simulink model "Demo_veDYNA_cs"  (Simulink 7.6)
settings: Solver=ode1  StartTime=0  StopTime=15  FixedStep=1/500  RelTol=1e-3
PreLoadFcn:
  | PreScanveDYNAPreLoadFcn(bdroot);
  | check_NUTS_defined;
  | 
  | assignin('base',['model_closed_' bdroot],false);
PostLoadFcn:
  | PreScanveDYNAPostLoadFcn(bdroot);
  | 
InitFcn:
  | vdy_SetExternalInputSource('ManLongCtrl',1,'Brake','other');
  | vdy_SetExternalInputSource('ManLongCtrl',1,'EngineTorque','other');
  | vdy_SetExternalInputSource('ManLatCtrl',1,'Steering','other');
  | 
  | PreScanveDYNAInitFcn(bdroot);
  | PreScanExperimentInitFcn(bdroot)
StopFcn:
  | PreScanExperimentStopFcn(bdroot)
undefined symbols (not defined in the file): at_period, CPT, vm_at_pulsewidth, vm_driver_dflt_gain, x_ini_VRML, y_ini_VRML, z_ini_VRML
libraries: dyna_cpt_lib x93, simulink x16, simulink_extras x14, PreScanSimulinkLibrary x6, anilib x3, dyna_lib x3, dyna_manctrl_lib x2, dyna_road_lib x2, PreScanUsefulBlocks x1, dyna_io_lib x1, dyna_demo_lib x1, dyna_usr_maneuver_states_lib x1
(part 8 of 8)

== system Demo_veDYNA_cs/Vedyna_Vehicle/CPT_MDL/MDL_SW/Driver/System Instance 1/lat_for_r_sw [1,..,4] ==
  Switch : Constant  Value=CPT.MDL_SW.Driver{1}.lat_for_r_sw.Switch.v
  Terminator : Terminator
  tag scope: Driver_1_lat_for_r_sw_SW=global
  wires:
  [Driver_1_lat_for_r_sw_SW] -> Terminator/1
  Switch/1 -> [Driver_1_lat_for_r_sw_SW]

== system Demo_veDYNA_cs/Vedyna_Vehicle/CPT_MDL/MDL_SW/Driver/System Instance 1/path_v_scale [1,..,4] ==
  Switch : Constant  Value=CPT.MDL_SW.Driver{1}.path_v_scale.Switch.v
  Terminator : Terminator
  tag scope: Driver_1_path_v_scale_SW=global
  wires:
  [Driver_1_path_v_scale_SW] -> Terminator/1
  Switch/1 -> [Driver_1_path_v_scale_SW]

== system Demo_veDYNA_cs/Vedyna_Vehicle/CPT_MDL/MDL_SW/Driver/System Instance 1/path_x_offset [1,..,4] ==
  Switch : Constant  Value=CPT.MDL_SW.Driver{1}.path_x_offset.Switch.v
  Terminator : Terminator
  tag scope: Driver_1_path_x_offset_SW=global
  wires:
  [Driver_1_path_x_offset_SW] -> Terminator/1
  Switch/1 -> [Driver_1_path_x_offset_SW]

== system Demo_veDYNA_cs/Vedyna_Vehicle/CPT_MDL/MDL_SW/Driver/System Instance 1/psi_path [1,..,4] ==
  Switch : Constant  Value=CPT.MDL_SW.Driver{1}.psi_path.Switch.v
  Terminator : Terminator
  tag scope: Driver_1_psi_path_SW=global
  wires:
  [Driver_1_psi_path_SW] -> Terminator/1
  Switch/1 -> [Driver_1_psi_path_SW]

== system Demo_veDYNA_cs/Vedyna_Vehicle/CPT_MDL/MDL_SW/Driver/System Instance 1/q_path [1,..,4] ==
  Switch : Constant  Value=CPT.MDL_SW.Driver{1}.q_path.Switch.v
  Terminator : Terminator
  tag scope: Driver_1_q_path_SW=global
  wires:
  [Driver_1_q_path_SW] -> Terminator/1
  Switch/1 -> [Driver_1_q_path_SW]

== system Demo_veDYNA_cs/Vedyna_Vehicle/CPT_MDL/MDL_SW/Driver/System Instance 1/rear_stiff [1,..,4] ==
  Switch : Constant  Value=CPT.MDL_SW.Driver{1}.rear_stiff.Switch.v
  Terminator : Terminator
  tag scope: Driver_1_rear_stiff_SW=global
  wires:
  [Driver_1_rear_stiff_SW] -> Terminator/1
  Switch/1 -> [Driver_1_rear_stiff_SW]

== system Demo_veDYNA_cs/Vedyna_Vehicle/CPT_MDL/MDL_SW/Driver/System Instance 1/rear_stiff_sw [1,..,4] ==
  Switch : Constant  Value=CPT.MDL_SW.Driver{1}.rear_stiff_sw.Switch.v
  Terminator : Terminator
  tag scope: Driver_1_rear_stiff_sw_SW=global
  wires:
  [Driver_1_rear_stiff_sw_SW] -> Terminator/1
  Switch/1 -> [Driver_1_rear_stiff_sw_SW]

== system Demo_veDYNA_cs/Vedyna_Vehicle/CPT_MDL/MDL_SW/Driver/System Instance 1/steer_max [1,..,4] ==
  Switch : Constant  Value=CPT.MDL_SW.Driver{1}.steer_max.Switch.v
  Terminator : Terminator
  tag scope: Driver_1_steer_max_SW=global
  wires:
  [Driver_1_steer_max_SW] -> Terminator/1
  Switch/1 -> [Driver_1_steer_max_SW]

== system Demo_veDYNA_cs/Vedyna_Vehicle/CPT_MDL/MDL_SW/Driver/System Instance 1/steer_min [1,..,4] ==
  Switch : Constant  Value=CPT.MDL_SW.Driver{1}.steer_min.Switch.v
  Terminator : Terminator
  tag scope: Driver_1_steer_min_SW=global
  wires:
  [Driver_1_steer_min_SW] -> Terminator/1
  Switch/1 -> [Driver_1_steer_min_SW]

== system Demo_veDYNA_cs/Vedyna_Vehicle/CPT_MDL/MDL_SW/Driver/System Instance 1/steer_rate_max [1,..,4] ==
  Switch : Constant  Value=CPT.MDL_SW.Driver{1}.steer_rate_max.Switch.v
  Terminator : Terminator
  tag scope: Driver_1_steer_rate_max_SW=global
  wires:
  [Driver_1_steer_rate_max_SW] -> Terminator/1
  Switch/1 -> [Driver_1_steer_rate_max_SW]

== system Demo_veDYNA_cs/Vedyna_Vehicle/CPT_MDL/MDL_SW/Driver/System Instance 1/steer_rate_min [1,..,4] ==
  Switch : Constant  Value=CPT.MDL_SW.Driver{1}.steer_rate_min.Switch.v
  Terminator : Terminator
  tag scope: Driver_1_steer_rate_min_SW=global
  wires:
  [Driver_1_steer_rate_min_SW] -> Terminator/1
  Switch/1 -> [Driver_1_steer_rate_min_SW]

== system Demo_veDYNA_cs/Vedyna_Vehicle/CPT_MDL/MDL_SW/Driver/System Instance 1/steer_smooth_t [1,..,4] ==
  Switch : Constant  Value=CPT.MDL_SW.Driver{1}.steer_smooth_t.Switch.v
  Terminator : Terminator
  tag scope: Driver_1_steer_smooth_t_SW=global
  wires:
  [Driver_1_steer_smooth_t_SW] -> Terminator/1
  Switch/1 -> [Driver_1_steer_smooth_t_SW]

== system Demo_veDYNA_cs/Vedyna_Vehicle/CPT_MDL/MDL_SW/Driver/System Instance 1/target_aim_x [1,..,4] ==
  Switch : Constant  Value=CPT.MDL_SW.Driver{1}.target_aim_x.Switch.v
  Terminator : Terminator
  tag scope: Driver_1_target_aim_x_SW=global
  wires:
  [Driver_1_target_aim_x_SW] -> Terminator/1
  Switch/1 -> [Driver_1_target_aim_x_SW]

== system Demo_veDYNA_cs/Vedyna_Vehicle/CPT_MDL/MDL_SW/Driver/System Instance 1/tgt_a_max [1,..,4] ==
  Switch : Constant  Value=CPT.MDL_SW.Driver{1}.tgt_a_max.Switch.v
  Terminator : Terminator
  tag scope: Driver_1_tgt_a_max_SW=global
  wires:
  [Driver_1_tgt_a_max_SW] -> Terminator/1
  Switch/1 -> [Driver_1_tgt_a_max_SW]

== system Demo_veDYNA_cs/Vedyna_Vehicle/CPT_MDL/MDL_SW/Driver/System Instance 1/tgt_acc_smooth_t [1,..,4] ==
  Switch : Constant  Value=CPT.MDL_SW.Driver{1}.tgt_acc_smooth_t.Switch.v
  Terminator : Terminator
  tag scope: Driver_1_tgt_acc_smooth_t_SW=global
  wires:
  [Driver_1_tgt_acc_smooth_t_SW] -> Terminator/1
  Switch/1 -> [Driver_1_tgt_acc_smooth_t_SW]

== system Demo_veDYNA_cs/Vedyna_Vehicle/CPT_MDL/MDL_SW/Driver/System Instance 1/tgt_ax_max [1,..,4] ==
  Switch : Constant  Value=CPT.MDL_SW.Driver{1}.tgt_ax_max.Switch.v
  Terminator : Terminator
  tag scope: Driver_1_tgt_ax_max_SW=global
  wires:
  [Driver_1_tgt_ax_max_SW] -> Terminator/1
  Switch/1 -> [Driver_1_tgt_ax_max_SW]

== system Demo_veDYNA_cs/Vedyna_Vehicle/CPT_MDL/MDL_SW/Driver/System Instance 1/tgt_ax_min [1,..,4] ==
  Switch : Constant  Value=CPT.MDL_SW.Driver{1}.tgt_ax_min.Switch.v
  Terminator : Terminator
  tag scope: Driver_1_tgt_ax_min_SW=global
  wires:
  [Driver_1_tgt_ax_min_SW] -> Terminator/1
  Switch/1 -> [Driver_1_tgt_ax_min_SW]

== system Demo_veDYNA_cs/Vedyna_Vehicle/CPT_MDL/MDL_SW/Driver/System Instance 1/tgt_ay_max [1,..,4] ==
  Switch : Constant  Value=CPT.MDL_SW.Driver{1}.tgt_ay_max.Switch.v
  Terminator : Terminator
  tag scope: Driver_1_tgt_ay_max_SW=global
  wires:
  [Driver_1_tgt_ay_max_SW] -> Terminator/1
  Switch/1 -> [Driver_1_tgt_ay_max_SW]

== system Demo_veDYNA_cs/Vedyna_Vehicle/CPT_MDL/MDL_SW/Driver/System Instance 1/tgt_v_max [1,..,4] ==
  Switch : Constant  Value=CPT.MDL_SW.Driver{1}.tgt_v_max.Switch.v
  Terminator : Terminator
  tag scope: Driver_1_tgt_v_max_SW=global
  wires:
  [Driver_1_tgt_v_max_SW] -> Terminator/1
  Switch/1 -> [Driver_1_tgt_v_max_SW]

== system Demo_veDYNA_cs/Vedyna_Vehicle/CPT_MDL/MDL_SW/Driver/System Instance 1/tgt_v_min [1,..,4] ==
  Switch : Constant  Value=CPT.MDL_SW.Driver{1}.tgt_v_min.Switch.v
  Terminator : Terminator
  tag scope: Driver_1_tgt_v_min_SW=global
  wires:
  [Driver_1_tgt_v_min_SW] -> Terminator/1
  Switch/1 -> [Driver_1_tgt_v_min_SW]

== system Demo_veDYNA_cs/Vedyna_Vehicle/CPT_MDL/MDL_SW/Driver/System Instance 1/use_simulink_sw [1,..,4] ==
  Switch : Constant  Value=CPT.MDL_SW.Driver{1}.use_simulink_sw.Switch.v
  Terminator : Terminator
  tag scope: Driver_1_use_simulink_sw_SW=global
  wires:
  [Driver_1_use_simulink_sw_SW] -> Terminator/1
  Switch/1 -> [Driver_1_use_simulink_sw_SW]

== system Demo_veDYNA_cs/Vedyna_Vehicle/CPT_MDL/MDL_SW/Driver/System Instance 1/v_comp_scale [1,..,4] ==
  Switch : Constant  Value=CPT.MDL_SW.Driver{1}.v_comp_scale.Switch.v
  Terminator : Terminator
  tag scope: Driver_1_v_comp_scale_SW=global
  wires:
  [Driver_1_v_comp_scale_SW] -> Terminator/1
  Switch/1 -> [Driver_1_v_comp_scale_SW]

== system Demo_veDYNA_cs/Vedyna_Vehicle/CPT_MDL/MDL_SW/Driver/System Instance 1/v_path [1,..,4] ==
  Switch : Constant  Value=CPT.MDL_SW.Driver{1}.v_path.Switch.v
  Terminator : Terminator
  tag scope: Driver_1_v_path_SW=global
  wires:
  [Driver_1_v_path_SW] -> Terminator/1
  Switch/1 -> [Driver_1_v_path_SW]

== system Demo_veDYNA_cs/Vedyna_Vehicle/CPT_MDL/MDL_SW/Engine/System Instance 1/ASR_Flag [1,..,4] ==
  Switch : Constant  Value=CPT.MDL_SW.Engine{1}.ASR_Flag.Switch.v
  Terminator : Terminator
  tag scope: Engine_1_ASR_Flag_SW=global
  wires:
  [Engine_1_ASR_Flag_SW] -> Terminator/1
  Switch/1 -> [Engine_1_ASR_Flag_SW]

== system Demo_veDYNA_cs/Vedyna_Vehicle/CPT_MDL/MDL_SW/Engine/System Instance 1/ASR_Torque [1,..,4] ==
  Switch : Constant  Value=CPT.MDL_SW.Engine{1}.ASR_Torque.Switch.v
  Terminator : Terminator
  tag scope: Engine_1_ASR_Torque_SW=global
  wires:
  [Engine_1_ASR_Torque_SW] -> Terminator/1
  Switch/1 -> [Engine_1_ASR_Torque_SW]

== system Demo_veDYNA_cs/Vedyna_Vehicle/CPT_MDL/MDL_SW/Engine/System Instance 1/HCI [1,..,n] ==
  Switch : Constant  Value=CPT.MDL_SW.Engine{1}.HCI.Switch.v
  Terminator : Terminator
  tag scope: Engine_1_HCI_SW=global
  wires:
  [Engine_1_HCI_SW] -> Terminator/1
  Switch/1 -> [Engine_1_HCI_SW]

== system Demo_veDYNA_cs/Vedyna_Vehicle/CPT_MDL/MDL_SW/Engine/System Instance 1/MSR_Flag [1,..,4] ==
  Switch : Constant  Value=CPT.MDL_SW.Engine{1}.MSR_Flag.Switch.v
  Terminator : Terminator
  tag scope: Engine_1_MSR_Flag_SW=global
  wires:
  [Engine_1_MSR_Flag_SW] -> Terminator/1
  Switch/1 -> [Engine_1_MSR_Flag_SW]

== system Demo_veDYNA_cs/Vedyna_Vehicle/CPT_MDL/MDL_SW/Engine/System Instance 1/MSR_Torque [1,..,4] ==
  Switch : Constant  Value=CPT.MDL_SW.Engine{1}.MSR_Torque.Switch.v
  Terminator : Terminator
  tag scope: Engine_1_MSR_Torque_SW=global
  wires:
  [Engine_1_MSR_Torque_SW] -> Terminator/1
  Switch/1 -> [Engine_1_MSR_Torque_SW]

== system Demo_veDYNA_cs/Vedyna_Vehicle/CPT_MDL/MDL_SW/GearCtrl/System Instance 1/Gear [1,..,4] ==
  Switch : Constant  Value=CPT.MDL_SW.GearCtrl{1}.Gear.Switch.v
  Terminator : Terminator
  tag scope: GearCtrl_1_Gear_SW=global
  wires:
  [GearCtrl_1_Gear_SW] -> Terminator/1
  Switch/1 -> [GearCtrl_1_Gear_SW]

== system Demo_veDYNA_cs/Vedyna_Vehicle/CPT_MDL/MDL_SW/GearCtrl/System Instance 1/GearMode [0,1] ==
  Switch : Constant  Value=CPT.MDL_SW.GearCtrl{1}.GearMode.Switch.v
  Terminator : Terminator
  tag scope: GearCtrl_1_GearMode_SW=global
  wires:
  [GearCtrl_1_GearMode_SW] -> Terminator/1
  Switch/1 -> [GearCtrl_1_GearMode_SW]

== system Demo_veDYNA_cs/Vedyna_Vehicle/CPT_MDL/MDL_SW/GearCtrl/System Instance 1/HCI [1,..,n] ==
  Switch : Constant  Value=CPT.MDL_SW.GearCtrl{1}.HCI.Switch.v
  Terminator : Terminator
  tag scope: GearCtrl_1_HCI_SW=global
  wires:
  [GearCtrl_1_HCI_SW] -> Terminator/1
  Switch/1 -> [GearCtrl_1_HCI_SW]

== system Demo_veDYNA_cs/Vedyna_Vehicle/CPT_MDL/MDL_SW/GearCtrl/System Instance 1/UpShiftRequest [1,..,4] ==
  Switch : Constant  Value=CPT.MDL_SW.GearCtrl{1}.UpShiftRequest.Switch.v
  Terminator : Terminator
  tag scope: GearCtrl_1_UpShiftRequest_SW=global
  wires:
  [GearCtrl_1_UpShiftRequest_SW] -> Terminator/1
  Switch/1 -> [GearCtrl_1_UpShiftRequest_SW]

== system Demo_veDYNA_cs/Vedyna_Vehicle/CPT_MDL/MDL_SW/ManLatCtrl/System Instance 1/Curvature [1,..,4] ==
  Switch : Constant  Value=CPT.MDL_SW.ManLatCtrl{1}.Curvature.Switch.v
  Terminator : Terminator
  tag scope: ManLatCtrl_1_Curvature_SW=global
  wires:
  [ManLatCtrl_1_Curvature_SW] -> Terminator/1
  Switch/1 -> [ManLatCtrl_1_Curvature_SW]

== system Demo_veDYNA_cs/Vedyna_Vehicle/CPT_MDL/MDL_SW/ManLatCtrl/System Instance 1/LatManMode [0,1,2] ==
  Switch : Constant  Value=CPT.MDL_SW.ManLatCtrl{1}.LatManMode.Switch.v
  Terminator : Terminator
  tag scope: ManLatCtrl_1_LatManMode_SW=global
  wires:
  [ManLatCtrl_1_LatManMode_SW] -> Terminator/1
  Switch/1 -> [ManLatCtrl_1_LatManMode_SW]

== system Demo_veDYNA_cs/Vedyna_Vehicle/CPT_MDL/MDL_SW/ManLatCtrl/System Instance 1/Steering [1,..,4] ==
  Switch : Constant  Value=CPT.MDL_SW.ManLatCtrl{1}.Steering.Switch.v
  Terminator : Terminator
  tag scope: ManLatCtrl_1_Steering_SW=global
  wires:
  [ManLatCtrl_1_Steering_SW] -> Terminator/1
  Switch/1 -> [ManLatCtrl_1_Steering_SW]

== system Demo_veDYNA_cs/Vedyna_Vehicle/CPT_MDL/MDL_SW/ManLongCtrl/System Instance 1/AccelerationY [1,..,4] ==
  Switch : Constant  Value=CPT.MDL_SW.ManLongCtrl{1}.AccelerationY.Switch.v
  Terminator : Terminator
  tag scope: ManLongCtrl_1_AccelerationY_SW=global
  wires:
  [ManLongCtrl_1_AccelerationY_SW] -> Terminator/1
  Switch/1 -> [ManLongCtrl_1_AccelerationY_SW]

== system Demo_veDYNA_cs/Vedyna_Vehicle/CPT_MDL/MDL_SW/ManLongCtrl/System Instance 1/Brake [1,..,4] ==
  Switch : Constant  Value=CPT.MDL_SW.ManLongCtrl{1}.Brake.Switch.v
  Terminator : Terminator
  tag scope: ManLongCtrl_1_Brake_SW=global
  wires:
  [ManLongCtrl_1_Brake_SW] -> Terminator/1
  Switch/1 -> [ManLongCtrl_1_Brake_SW]

== system Demo_veDYNA_cs/Vedyna_Vehicle/CPT_MDL/MDL_SW/ManLongCtrl/System Instance 1/EngineTorque [1,..,4] ==
  Switch : Constant  Value=CPT.MDL_SW.ManLongCtrl{1}.EngineTorque.Switch.v
  Terminator : Terminator
  tag scope: ManLongCtrl_1_EngineTorque_SW=global
  wires:
  [ManLongCtrl_1_EngineTorque_SW] -> Terminator/1
  Switch/1 -> [ManLongCtrl_1_EngineTorque_SW]

== system Demo_veDYNA_cs/Vedyna_Vehicle/CPT_MDL/MDL_SW/ManLongCtrl/System Instance 1/LongManMode [0,1,2] ==
  Switch : Constant  Value=CPT.MDL_SW.ManLongCtrl{1}.LongManMode.Switch.v
  Terminator : Terminator
  tag scope: ManLongCtrl_1_LongManMode_SW=global
  wires:
  [ManLongCtrl_1_LongManMode_SW] -> Terminator/1
  Switch/1 -> [ManLongCtrl_1_LongManMode_SW]

== system Demo_veDYNA_cs/Vedyna_Vehicle/CPT_MDL/MDL_SW/ManLongCtrl/System Instance 1/Speed [1,..,4] ==
  Switch : Constant  Value=CPT.MDL_SW.ManLongCtrl{1}.Speed.Switch.v
  Terminator : Terminator
  tag scope: ManLongCtrl_1_Speed_SW=global
  wires:
  [ManLongCtrl_1_Speed_SW] -> Terminator/1
  Switch/1 -> [ManLongCtrl_1_Speed_SW]

== system Demo_veDYNA_cs/Vedyna_Vehicle/CPT_MDL/MDL_SW/ManLongCtrl/System Instance 1/Throttle [1,..,4] ==
  Switch : Constant  Value=CPT.MDL_SW.ManLongCtrl{1}.Throttle.Switch.v
  Terminator : Terminator
  tag scope: ManLongCtrl_1_Throttle_SW=global
  wires:
  [ManLongCtrl_1_Throttle_SW] -> Terminator/1
  Switch/1 -> [ManLongCtrl_1_Throttle_SW]

== system Demo_veDYNA_cs/Vedyna_Vehicle/CPT_MDL/MDL_SW/ManSchedule/System Instance 1/HCI [1,..,n] ==
  Switch : Constant  Value=CPT.MDL_SW.ManSchedule{1}.HCI.Switch.v
  Terminator : Terminator
  tag scope: ManSchedule_1_HCI_SW=global
  wires:
  [ManSchedule_1_HCI_SW] -> Terminator/1
  Switch/1 -> [ManSchedule_1_HCI_SW]

== system Demo_veDYNA_cs/Vedyna_Vehicle/CPT_MDL/MDL_SW/ManSchedule/System Instance 2/HCI [1,..,n] ==
  Switch : Constant  Value=CPT.MDL_SW.ManSchedule{2}.HCI.Switch.v
  Terminator : Terminator
  tag scope: ManSchedule_2_HCI_SW=global
  wires:
  [ManSchedule_2_HCI_SW] -> Terminator/1
  Switch/1 -> [ManSchedule_2_HCI_SW]

== system Demo_veDYNA_cs/Vedyna_Vehicle/CPT_MDL/MDL_SW/ManSchedule/System Instance 3/HCI [1,..,n] ==
  Switch : Constant  Value=CPT.MDL_SW.ManSchedule{3}.HCI.Switch.v
  Terminator : Terminator
  tag scope: ManSchedule_3_HCI_SW=global
  wires:
  [ManSchedule_3_HCI_SW] -> Terminator/1
  Switch/1 -> [ManSchedule_3_HCI_SW]

== system Demo_veDYNA_cs/Vedyna_Vehicle/CPT_MDL/MDL_SW/Road/System Instance 1/HCI [1,..,n] ==
  Switch : Constant  Value=CPT.MDL_SW.Road{1}.HCI.Switch.v
  Terminator : Terminator
  tag scope: Road_1_HCI_SW=global
  wires:
  [Road_1_HCI_SW] -> Terminator/1
  Switch/1 -> [Road_1_HCI_SW]

== system Demo_veDYNA_cs/Vedyna_Vehicle/CPT_MDL/MDL_SW/Simctrl/System Instance 1/Reset [0,1] ==
  Switch : Constant  Value=CPT.MDL_SW.Simctrl{1}.Reset.Switch.v
  Terminator : Terminator
  tag scope: Simctrl_1_Reset_SW=global
  wires:
  [Simctrl_1_Reset_SW] -> Terminator/1
  Switch/1 -> [Simctrl_1_Reset_SW]

== system Demo_veDYNA_cs/Vedyna_Vehicle/CPT_MDL/MDL_SW/Simctrl/System Instance 1/Suspend [0,1] ==
  Switch : Constant  Value=CPT.MDL_SW.Simctrl{1}.Suspend.Switch.v
  Terminator : Terminator
  tag scope: Simctrl_1_Suspend_SW=global
  wires:
  [Simctrl_1_Suspend_SW] -> Terminator/1
  Switch/1 -> [Simctrl_1_Suspend_SW]

== system Demo_veDYNA_cs/Vedyna_Vehicle/CPT_MDL/MDL_SW/Tmeasy/System Instance 1/HCI [1,..,n] ==
  Switch : Constant  Value=CPT.MDL_SW.Tmeasy{1}.HCI.Switch.v
  Terminator : Terminator
  tag scope: Tmeasy_1_HCI_SW=global
  wires:
  [Tmeasy_1_HCI_SW] -> Terminator/1
  Switch/1 -> [Tmeasy_1_HCI_SW]

== system Demo_veDYNA_cs/Vedyna_Vehicle/CPT_MDL/MDL_SW/Tmeasy/System Instance 1/RoadMueScale [1,..,4] ==
  Switch : Constant  Value=CPT.MDL_SW.Tmeasy{1}.RoadMueScale.Switch.v
  Terminator : Terminator
  tag scope: Tmeasy_1_RoadMueScale_SW=global
  wires:
  [Tmeasy_1_RoadMueScale_SW] -> Terminator/1
  Switch/1 -> [Tmeasy_1_RoadMueScale_SW]

== system Demo_veDYNA_cs/Vedyna_Vehicle/CPT_MDL/MDL_SW/Tmeasy/System Instance 2/HCI [1,..,n] ==
  Switch : Constant  Value=CPT.MDL_SW.Tmeasy{2}.HCI.Switch.v
  Terminator : Terminator
  tag scope: Tmeasy_2_HCI_SW=global
  wires:
  [Tmeasy_2_HCI_SW] -> Terminator/1
  Switch/1 -> [Tmeasy_2_HCI_SW]

== system Demo_veDYNA_cs/Vedyna_Vehicle/CPT_MDL/MDL_SW/Tmeasy/System Instance 2/RoadMueScale [1,..,4] ==
  Switch : Constant  Value=CPT.MDL_SW.Tmeasy{2}.RoadMueScale.Switch.v
  Terminator : Terminator
  tag scope: Tmeasy_2_RoadMueScale_SW=global
  wires:
  [Tmeasy_2_RoadMueScale_SW] -> Terminator/1
  Switch/1 -> [Tmeasy_2_RoadMueScale_SW]

== system Demo_veDYNA_cs/Vedyna_Vehicle/CPT_MDL/MDL_SW/Tmeasy/System Instance 3/HCI [1,..,n] ==
  Switch : Constant  Value=CPT.MDL_SW.Tmeasy{3}.HCI.Switch.v
  Terminator : Terminator
  tag scope: Tmeasy_3_HCI_SW=global
  wires:
  [Tmeasy_3_HCI_SW] -> Terminator/1
  Switch/1 -> [Tmeasy_3_HCI_SW]

== system Demo_veDYNA_cs/Vedyna_Vehicle/CPT_MDL/MDL_SW/Tmeasy/System Instance 3/RoadMueScale [1,..,4] ==
  Switch : Constant  Value=CPT.MDL_SW.Tmeasy{3}.RoadMueScale.Switch.v
  Terminator : Terminator
  tag scope: Tmeasy_3_RoadMueScale_SW=global
  wires:
  [Tmeasy_3_RoadMueScale_SW] -> Terminator/1
  Switch/1 -> [Tmeasy_3_RoadMueScale_SW]

== system Demo_veDYNA_cs/Vedyna_Vehicle/CPT_MDL/MDL_SW/Tmeasy/System Instance 4/HCI [1,..,n] ==
  Switch : Constant  Value=CPT.MDL_SW.Tmeasy{4}.HCI.Switch.v
  Terminator : Terminator
  tag scope: Tmeasy_4_HCI_SW=global
  wires:
  [Tmeasy_4_HCI_SW] -> Terminator/1
  Switch/1 -> [Tmeasy_4_HCI_SW]

== system Demo_veDYNA_cs/Vedyna_Vehicle/CPT_MDL/MDL_SW/Tmeasy/System Instance 4/RoadMueScale [1,..,4] ==
  Switch : Constant  Value=CPT.MDL_SW.Tmeasy{4}.RoadMueScale.Switch.v
  Terminator : Terminator
  tag scope: Tmeasy_4_RoadMueScale_SW=global
  wires:
  [Tmeasy_4_RoadMueScale_SW] -> Terminator/1
  Switch/1 -> [Tmeasy_4_RoadMueScale_SW]

== system Demo_veDYNA_cs/Vedyna_Vehicle/CPT_MDL/MDL_SW/Tmeasy/System Instance 5/HCI [1,..,n] ==
  Switch : Constant  Value=CPT.MDL_SW.Tmeasy{5}.HCI.Switch.v
  Terminator : Terminator
  tag scope: Tmeasy_5_HCI_SW=global
  wires:
  [Tmeasy_5_HCI_SW] -> Terminator/1
  Switch/1 -> [Tmeasy_5_HCI_SW]

== system Demo_veDYNA_cs/Vedyna_Vehicle/CPT_MDL/MDL_SW/Tmeasy/System Instance 5/RoadMueScale [1,..,4] ==
  Switch : Constant  Value=CPT.MDL_SW.Tmeasy{5}.RoadMueScale.Switch.v
  Terminator : Terminator
  tag scope: Tmeasy_5_RoadMueScale_SW=global
  wires:
  [Tmeasy_5_RoadMueScale_SW] -> Terminator/1
  Switch/1 -> [Tmeasy_5_RoadMueScale_SW]

== system Demo_veDYNA_cs/Vedyna_Vehicle/CPT_MDL/MDL_SW/Tmeasy/System Instance 6/HCI [1,..,n] ==
  Switch : Constant  Value=CPT.MDL_SW.Tmeasy{6}.HCI.Switch.v
  Terminator : Terminator
  tag scope: Tmeasy_6_HCI_SW=global
  wires:
  [Tmeasy_6_HCI_SW] -> Terminator/1
  Switch/1 -> [Tmeasy_6_HCI_SW]

== system Demo_veDYNA_cs/Vedyna_Vehicle/CPT_MDL/MDL_SW/Tmeasy/System Instance 6/RoadMueScale [1,..,4] ==
  Switch : Constant  Value=CPT.MDL_SW.Tmeasy{6}.RoadMueScale.Switch.v
  Terminator : Terminator
  tag scope: Tmeasy_6_RoadMueScale_SW=global
  wires:
  [Tmeasy_6_RoadMueScale_SW] -> Terminator/1
  Switch/1 -> [Tmeasy_6_RoadMueScale_SW]

== system Demo_veDYNA_cs/Vedyna_Vehicle/CPT_MDL/MDL_SW/Tmeasy/System Instance 7/HCI [1,..,n] ==
  Switch : Constant  Value=CPT.MDL_SW.Tmeasy{7}.HCI.Switch.v
  Terminator : Terminator
  tag scope: Tmeasy_7_HCI_SW=global
  wires:
  Switch/1 -> [Tmeasy_7_HCI_SW]
  [Tmeasy_7_HCI_SW] -> Terminator/1

== system Demo_veDYNA_cs/Vedyna_Vehicle/CPT_MDL/MDL_SW/Tmeasy/System Instance 7/RoadMueScale [1,..,4] ==
  Switch : Constant  Value=CPT.MDL_SW.Tmeasy{7}.RoadMueScale.Switch.v
  Terminator : Terminator
  tag scope: Tmeasy_7_RoadMueScale_SW=global
  wires:
  Switch/1 -> [Tmeasy_7_RoadMueScale_SW]
  [Tmeasy_7_RoadMueScale_SW] -> Terminator/1

== system Demo_veDYNA_cs/Vedyna_Vehicle/CPT_MDL/MDL_SW/Tmeasy/System Instance 8/HCI [1,..,n] ==
  Switch : Constant  Value=CPT.MDL_SW.Tmeasy{8}.HCI.Switch.v
  Terminator : Terminator
  tag scope: Tmeasy_8_HCI_SW=global
  wires:
  Switch/1 -> [Tmeasy_8_HCI_SW]
  [Tmeasy_8_HCI_SW] -> Terminator/1

== system Demo_veDYNA_cs/Vedyna_Vehicle/CPT_MDL/MDL_SW/Tmeasy/System Instance 8/RoadMueScale [1,..,4] ==
  Switch : Constant  Value=CPT.MDL_SW.Tmeasy{8}.RoadMueScale.Switch.v
  Terminator : Terminator
  tag scope: Tmeasy_8_RoadMueScale_SW=global
  wires:
  Switch/1 -> [Tmeasy_8_RoadMueScale_SW]
  [Tmeasy_8_RoadMueScale_SW] -> Terminator/1

== system Demo_veDYNA_cs/Vedyna_Vehicle/CPT_MDL/MDL_SW/Vehicle/System Instance 1/HCI [1,..,n] ==
  Switch : Constant  Value=CPT.MDL_SW.Vehicle{1}.HCI.Switch.v
  Terminator : Terminator
  tag scope: Vehicle_1_HCI_SW=global
  wires:
  [Vehicle_1_HCI_SW] -> Terminator/1
  Switch/1 -> [Vehicle_1_HCI_SW]

== system Demo_veDYNA_cs/Vedyna_Vehicle/CPT_MDL/MDL_SW/Wheel/System Instance 1/HCI [1,..,n] ==
  Switch : Constant  Value=CPT.MDL_SW.Wheel{1}.HCI.Switch.v
  Terminator : Terminator
  tag scope: Wheel_1_HCI_SW=global
  wires:
  [Wheel_1_HCI_SW] -> Terminator/1
  Switch/1 -> [Wheel_1_HCI_SW]

== system Demo_veDYNA_cs/Vedyna_Vehicle/CPT_MDL/MDL_SW/Wheel/System Instance 1/pbrm [1,..,4] ==
  Switch : Constant  Value=CPT.MDL_SW.Wheel{1}.pbrm.Switch.v
  Terminator : Terminator
  tag scope: Wheel_1_pbrm_SW=global
  wires:
  [Wheel_1_pbrm_SW] -> Terminator/1
  Switch/1 -> [Wheel_1_pbrm_SW]

== system Demo_veDYNA_cs/Vedyna_Vehicle/CPT_MDL/MDL_SW/Wheel/System Instance 2/HCI [1,..,n] ==
  Switch : Constant  Value=CPT.MDL_SW.Wheel{2}.HCI.Switch.v
  Terminator : Terminator
  tag scope: Wheel_2_HCI_SW=global
  wires:
  [Wheel_2_HCI_SW] -> Terminator/1
  Switch/1 -> [Wheel_2_HCI_SW]

== system Demo_veDYNA_cs/Vedyna_Vehicle/CPT_MDL/MDL_SW/Wheel/System Instance 2/pbrm [1,..,4] ==
  Switch : Constant  Value=CPT.MDL_SW.Wheel{2}.pbrm.Switch.v
  Terminator : Terminator
  tag scope: Wheel_2_pbrm_SW=global
  wires:
  [Wheel_2_pbrm_SW] -> Terminator/1
  Switch/1 -> [Wheel_2_pbrm_SW]

== system Demo_veDYNA_cs/Vedyna_Vehicle/CPT_MDL/MDL_SW/Wheel/System Instance 3/HCI [1,..,n] ==
  Switch : Constant  Value=CPT.MDL_SW.Wheel{3}.HCI.Switch.v
  Terminator : Terminator
  tag scope: Wheel_3_HCI_SW=global
  wires:
  [Wheel_3_HCI_SW] -> Terminator/1
  Switch/1 -> [Wheel_3_HCI_SW]

== system Demo_veDYNA_cs/Vedyna_Vehicle/CPT_MDL/MDL_SW/Wheel/System Instance 3/pbrm [1,..,4] ==
  Switch : Constant  Value=CPT.MDL_SW.Wheel{3}.pbrm.Switch.v
  Terminator : Terminator
  tag scope: Wheel_3_pbrm_SW=global
  wires:
  [Wheel_3_pbrm_SW] -> Terminator/1
  Switch/1 -> [Wheel_3_pbrm_SW]

== system Demo_veDYNA_cs/Vedyna_Vehicle/CPT_MDL/MDL_SW/Wheel/System Instance 4/HCI [1,..,n] ==
  Switch : Constant  Value=CPT.MDL_SW.Wheel{4}.HCI.Switch.v
  Terminator : Terminator
  tag scope: Wheel_4_HCI_SW=global
  wires:
  [Wheel_4_HCI_SW] -> Terminator/1
  Switch/1 -> [Wheel_4_HCI_SW]

== system Demo_veDYNA_cs/Vedyna_Vehicle/CPT_MDL/MDL_SW/Wheel/System Instance 4/pbrm [1,..,4] ==
  Switch : Constant  Value=CPT.MDL_SW.Wheel{4}.pbrm.Switch.v
  Terminator : Terminator
  tag scope: Wheel_4_pbrm_SW=global
  wires:
  [Wheel_4_pbrm_SW] -> Terminator/1
  Switch/1 -> [Wheel_4_pbrm_SW]

== system Demo_veDYNA_cs/Vedyna_Vehicle/CPT_MDL/MDL_SW/Wheel/System Instance 5/HCI [1,..,n] ==
  Switch : Constant  Value=CPT.MDL_SW.Wheel{5}.HCI.Switch.v
  Terminator : Terminator
  tag scope: Wheel_5_HCI_SW=global
  wires:
  [Wheel_5_HCI_SW] -> Terminator/1
  Switch/1 -> [Wheel_5_HCI_SW]

== system Demo_veDYNA_cs/Vedyna_Vehicle/CPT_MDL/MDL_SW/Wheel/System Instance 5/pbrm [1,..,4] ==
  Switch : Constant  Value=CPT.MDL_SW.Wheel{5}.pbrm.Switch.v
  Terminator : Terminator
  tag scope: Wheel_5_pbrm_SW=global
  wires:
  [Wheel_5_pbrm_SW] -> Terminator/1
  Switch/1 -> [Wheel_5_pbrm_SW]

== system Demo_veDYNA_cs/Vedyna_Vehicle/CPT_MDL/MDL_SW/Wheel/System Instance 6/HCI [1,..,n] ==
  Switch : Constant  Value=CPT.MDL_SW.Wheel{6}.HCI.Switch.v
  Terminator : Terminator
  tag scope: Wheel_6_HCI_SW=global
  wires:
  [Wheel_6_HCI_SW] -> Terminator/1
  Switch/1 -> [Wheel_6_HCI_SW]

== system Demo_veDYNA_cs/Vedyna_Vehicle/CPT_MDL/MDL_SW/Wheel/System Instance 6/pbrm [1,..,4] ==
  Switch : Constant  Value=CPT.MDL_SW.Wheel{6}.pbrm.Switch.v
  Terminator : Terminator
  tag scope: Wheel_6_pbrm_SW=global
  wires:
  [Wheel_6_pbrm_SW] -> Terminator/1
  Switch/1 -> [Wheel_6_pbrm_SW]

== system Demo_veDYNA_cs/Vedyna_Vehicle/CPT_MDL/MDL_SW/Wheel/System Instance 7/HCI [1,..,n] ==
  Switch : Constant  Value=CPT.MDL_SW.Wheel{7}.HCI.Switch.v
  Terminator : Terminator
  tag scope: Wheel_7_HCI_SW=global
  wires:
  Switch/1 -> [Wheel_7_HCI_SW]
  [Wheel_7_HCI_SW] -> Terminator/1

== system Demo_veDYNA_cs/Vedyna_Vehicle/CPT_MDL/MDL_SW/Wheel/System Instance 7/pbrm [1,..,4] ==
  Switch : Constant  Value=CPT.MDL_SW.Wheel{7}.pbrm.Switch.v
  Terminator : Terminator
  tag scope: Wheel_7_pbrm_SW=global
  wires:
  Switch/1 -> [Wheel_7_pbrm_SW]
  [Wheel_7_pbrm_SW] -> Terminator/1

== system Demo_veDYNA_cs/Vedyna_Vehicle/CPT_MDL/MDL_SW/Wheel/System Instance 8/HCI [1,..,n] ==
  Switch : Constant  Value=CPT.MDL_SW.Wheel{8}.HCI.Switch.v
  Terminator : Terminator
  tag scope: Wheel_8_HCI_SW=global
  wires:
  Switch/1 -> [Wheel_8_HCI_SW]
  [Wheel_8_HCI_SW] -> Terminator/1

== system Demo_veDYNA_cs/Vedyna_Vehicle/CPT_MDL/MDL_SW/Wheel/System Instance 8/pbrm [1,..,4] ==
  Switch : Constant  Value=CPT.MDL_SW.Wheel{8}.pbrm.Switch.v
  Terminator : Terminator
  tag scope: Wheel_8_pbrm_SW=global
  wires:
  Switch/1 -> [Wheel_8_pbrm_SW]
  [Wheel_8_pbrm_SW] -> Terminator/1

== system Demo_veDYNA_cs/Vedyna_Vehicle/vdy_mdl/Vehicle System/veDYNA Vehicle Subsystem/Brake System/Configurable Subsystem ==
  Brake Pedal Position : Inport
  I/O Vector : Inport  Port=2
  SyncIn : Inport  Port=3
  HCI Switch : Inport  Port=4
  veDYNA Brake Hydraulics : dyna_brakehydraulics_lib/veDYNA Brake Hydraulics  Tag=vedynaBrkHydMask  local_comp_inst=1  system_comp_inst=1
  SyncOut : Outport
  BrkHyd Info : Outport  Port=2
  Master Cylinder Pressure : Outport  Port=3
  Wheel 1 Cylinder Pressure : Outport  Port=4
  Wheel 2 Cylinder Pressure : Outport  Port=5
  Wheel 3 Cylinder Pressure : Outport  Port=6
  Wheel 4 Cylinder Pressure : Outport  Port=7
  Wheel 5 Cylinder Pressure : Outport  Port=8
  Wheel 6 Cylinder Pressure : Outport  Port=9
  Wheel 7 Cylinder Pressure : Outport  Port=10
  Wheel 8 Cylinder Pressure : Outport  Port=11
  wires:
  veDYNA Brake Hydraulics/11 -> Wheel 8 Cylinder Pressure/1
  veDYNA Brake Hydraulics/10 -> Wheel 7 Cylinder Pressure/1
  veDYNA Brake Hydraulics/9 -> Wheel 6 Cylinder Pressure/1
  veDYNA Brake Hydraulics/8 -> Wheel 5 Cylinder Pressure/1
  veDYNA Brake Hydraulics/7 -> Wheel 4 Cylinder Pressure/1
  veDYNA Brake Hydraulics/6 -> Wheel 3 Cylinder Pressure/1
  veDYNA Brake Hydraulics/5 -> Wheel 2 Cylinder Pressure/1
  veDYNA Brake Hydraulics/4 -> Wheel 1 Cylinder Pressure/1
  veDYNA Brake Hydraulics/3 -> Master Cylinder Pressure/1
  veDYNA Brake Hydraulics/2 -> BrkHyd Info/1
  veDYNA Brake Hydraulics/1 -> SyncOut/1
  HCI Switch/1 -> veDYNA Brake Hydraulics/4
  SyncIn/1 -> veDYNA Brake Hydraulics/3
  I/O Vector/1 -> veDYNA Brake Hydraulics/2
  Brake Pedal Position/1 -> veDYNA Brake Hydraulics/1

== system Demo_veDYNA_cs/Vedyna_Vehicle/vdy_mdl/Vehicle System/veDYNA Vehicle Subsystem/Brake System/HCI Switch ==
  SW_BrkHyd_1_HCI : dyna_cpt_lib/CPT_MDL_HCI_SW_ACCESS  Tag=vedynaCPT_MDL_HCI_SW_ACCESS  component=BrkHyd  system_inst=1  parameter=HCI
  HCI Switch : Outport
  wires:
  SW_BrkHyd_1_HCI/1 -> HCI Switch/1

== system Demo_veDYNA_cs/Vedyna_Vehicle/vdy_mdl/Vehicle System/veDYNA Vehicle Subsystem/External Vehicle Inputs (from I/O)/Inputs from I/O ==
  I/O Vector : Inport
  Demux1 : Demux  Outputs=[1,1,1,1]
  ASR Flag : Outport
  ASR Torque : Outport  Port=2
  MSR Flag : Outport  Port=3
  MSR Torque : Outport  Port=4
  wires:
  I/O Vector/1 -> Demux1/1
  Demux1/1 -> ASR Flag/1
  Demux1/2 -> ASR Torque/1
  Demux1/3 -> MSR Flag/1
  Demux1/4 -> MSR Torque/1

== system Demo_veDYNA_cs/Vedyna_Vehicle/vdy_mdl/Vehicle System/veDYNA Vehicle Subsystem/External Vehicle Inputs (from I/O)/Inputs from Maneuver ==
  Maneuver Commands : Inport
  Demux1 : Demux  Outputs=[1,1,1,1,1,1,1,1,1]
  Road mue Wheel 1 : Outport
  Road mue Wheel 2 : Outport  Port=2
  Road mue Wheel 3 : Outport  Port=3
  Road mue Wheel 4 : Outport  Port=4
  Road mue Wheel 5 : Outport  Port=5
  Road mue Wheel 6 : Outport  Port=6
  Hydropulse Flag : Outport  Port=7
  Hydropulse Left (Wheels 1,3,5) : Outport  Port=8
  Hydropulse Right (Wheels 2,4,6) : Outport  Port=9
  wires:
  Demux1/1 -> Road mue Wheel 1/1
  Demux1/2 -> Road mue Wheel 2/1
  Demux1/3 -> Road mue Wheel 3/1
  Demux1/4 -> Road mue Wheel 4/1
  Demux1/5 -> Road mue Wheel 5/1
  Demux1/6 -> Road mue Wheel 6/1
  Demux1/7 -> Hydropulse Flag/1
  Demux1/8 -> Hydropulse Left (Wheels 1,3,5)/1
  Demux1/9 -> Hydropulse Right (Wheels 2,4,6)/1
  Maneuver Commands/1 -> Demux1/1
